simulink model "PcontrollerModel2018"  (R2020a)
settings: Solver=ode45  StartTime=0.0  StopTime=t_sim  RelTol=1e-5
undefined symbols (not defined in the file): A1, A2, du, g, h10, h20, k, Kh, Ki, Km, Kr, Kv, qu0, t_step, Tv, uh0
settings Model: Creator=Mislav  LastModifiedBy=Mislav
settings DataIOCC: ReturnWorkspaceOutputs=off
settings DebuggingCC: ArithmeticOperatorsInVariantConditions=warning
settings SFSimCC: CustomCodeUndefinedFunction=UseInterfaceOnly

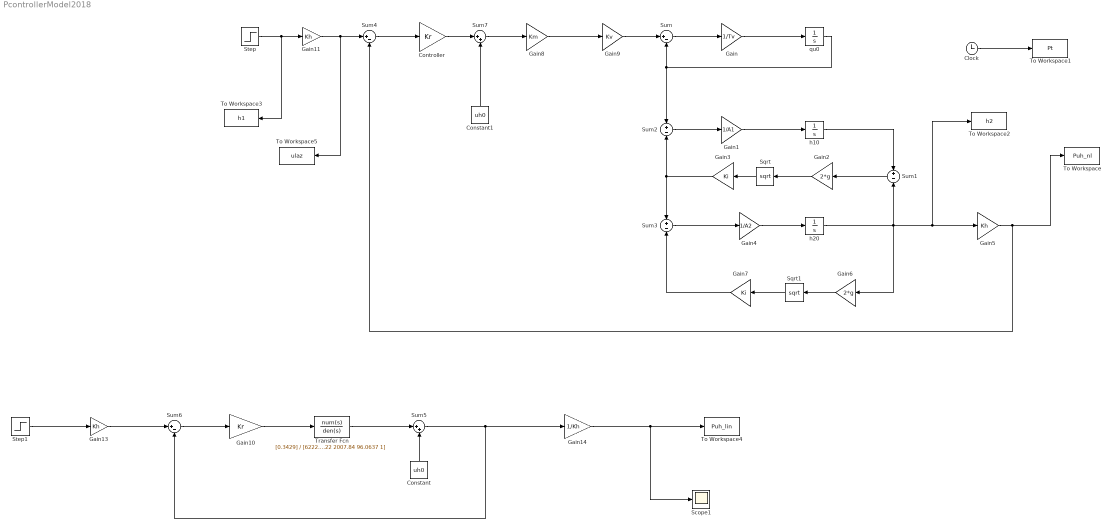
== system PcontrollerModel2018 ==
  Clock : Clock
  Constant : Constant  Value=uh0
  Constant1 : Constant  Value=uh0
  Controller : Gain  Gain=Kr
  Gain : Gain  Gain=1/Tv
  Gain1 : Gain  Gain=1/A1
  Gain10 : Gain  Gain=Kr
  Gain11 : Gain  Gain=Kh
  Gain13 : Gain  Gain=Kh
  Gain14 : Gain  Gain=1/Kh
  Gain2 : Gain  Gain=2*g
  Gain3 : Gain  Gain=Ki
  Gain4 : Gain  Gain=1/A2
  Gain5 : Gain  Gain=Kh
  Gain6 : Gain  Gain=2*g
  Gain7 : Gain  Gain=Ki
  Gain8 : Gain  Gain=Km
  Gain9 : Gain  Gain=Kv
  Scope1 : Scope
  Sqrt : Sqrt  SaturateOnIntegerOverflow=on
  Sqrt1 : Sqrt  SaturateOnIntegerOverflow=on
  Step : Step  Time=t_step  After=h20*1.1  SampleTime=0
  Step1 : Step  Time=t_step  After=k*du  SampleTime=0
  Sum : Sum  Inputs=|+-
  Sum1 : Sum  Inputs=+-
  Sum2 : Sum  Inputs=+|-
  Sum3 : Sum  Inputs=+|-
  Sum4 : Sum  Inputs=|+-
  Sum5 : Sum  Inputs=|++
  Sum6 : Sum  Inputs=|+-
  Sum7 : Sum  Inputs=|++
  To Workspace : ToWorkspace  VariableName=Puh_nl  SampleTime=-1
      settings: Save2DSignal=2-D array (concatenate along first dimension)
  To Workspace1 : ToWorkspace  VariableName=Pt  SampleTime=-1
      settings: Save2DSignal=2-D array (concatenate along first dimension)
  To Workspace2 : ToWorkspace  VariableName=h2  SampleTime=-1
      settings: Save2DSignal=2-D array (concatenate along first dimension)
  To Workspace3 : ToWorkspace  VariableName=h1  SampleTime=-1
      settings: Save2DSignal=2-D array (concatenate along first dimension)
  To Workspace4 : ToWorkspace  VariableName=Puh_lin  SampleTime=-1
      settings: Save2DSignal=2-D array (concatenate along first dimension)
  To Workspace5 : ToWorkspace  VariableName=ulaz  SampleTime=-1
      settings: Save2DSignal=2-D array (concatenate along first dimension)
  Transfer Fcn : TransferFcn  Numerator=[0.3429]  Denominator=[6222.22 2007.84 96.0637 1]
  "h10 " : Integrator  InitialCondition=h10
  "h20 " : Integrator  InitialCondition=h20
  "qu0 " : Integrator  InitialCondition=qu0
  wires:
  Gain10/1 -> Transfer Fcn/1
  Constant1/1 -> Sum7/2
  Sqrt/1 -> Gain3/1
  Sum2/1 -> Gain1/1
  Gain5/1 -> To Workspace/1, Sum4/2
  Sum5/1 -> Gain14/1, Sum6/2
  "h20 "/1 -> Gain6/1, To Workspace2/1, Gain5/1, Sum1/2
  Step/1 -> To Workspace3/1, Gain11/1
  Gain13/1 -> Sum6/1
  Sum7/1 -> Gain8/1
  "qu0 "/1 -> Sum/2, Sum2/1
  Step1/1 -> Gain13/1
  Gain14/1 -> Scope1/1, To Workspace4/1
  Sum1/1 -> Gain2/1
  Gain11/1 -> To Workspace5/1, Sum4/1
  Gain2/1 -> Sqrt/1
  Clock/1 -> To Workspace1/1
  Gain4/1 -> "h20 "/1
  Sum6/1 -> Gain10/1
  Constant/1 -> Sum5/2
  Gain7/1 -> Sum3/2
  Gain3/1 -> Sum2/2, Sum3/1
  Transfer Fcn/1 -> Sum5/1
  Gain/1 -> "qu0 "/1
  Controller/1 -> Sum7/1
  "h10 "/1 -> Sum1/1
  Gain6/1 -> Sqrt1/1
  Sum3/1 -> Gain4/1
  Gain8/1 -> Gain9/1
  Sum4/1 -> Controller/1
  Gain1/1 -> "h10 "/1
  Sum/1 -> Gain/1
  Sqrt1/1 -> Gain7/1
  Gain9/1 -> Sum/1
